simulink library "utility_service_lib"  (Simulink 8.1)
settings: Solver=ode45  StartTime=0.0  StopTime=10.0  RelTol=1e-3
undefined symbols (not defined in the file or in its folder): cable_spec, Left, Ts, type, V
libraries: cables_lib x6, breaker_lib x4, artemis x3, transformer_lib x2, rtlab x1, ssn_lib x1, powerlib x1
settings Model: Creator=RE25624  LastModifiedBy=re25624

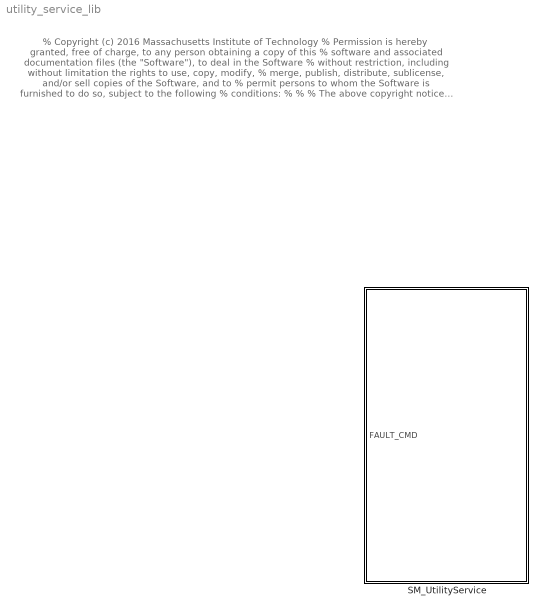
== system utility_service_lib ==
  note: % Copyright (c) 2016 Massachusetts Institute of Technology
      | % Permission is hereby granted, free of charge, to any person obtaining a copy of this
      | % software and associated documentation files (the "Software"), to deal in the Software
      | % without restriction, including without limitation the rights to use, copy, modify,
      | % merge, publish, distribute, sublicense, and/or sell copies of the Software, and to
      | % permit persons to whom the Software is furnished to do so, subject to the following
      | % conditions:
      | %
      | %
      | % The above copyright notice and this permission notice shall be included in
      | % all copies or substantial portions of the Software.
      | %
      | % THE SOFTWARE IS PROVIDED "AS IS", WITHOUT WARRANTY OF ANY KIND, EXPRESS OR IMPLIED,
      | % INCLUDING BUT NOT LIMITED TO THE WARRANTIES OF MERCHANTABILITY, FITNESS FOR A
      | % PARTICULAR PURPOSE AND NONINFRINGEMENT. IN NO EVENT SHALL THE AUTHORS OR COPYRIGHT
      | % HOLDERS BE LIABLE FOR ANY CLAIM, DAMAGES OR OTHER LIABILITY, WHETHER IN AN ACTION
      | % OF CONTRACT, TORT OR OTHERWISE, ARISING FROM, OUT OF OR IN CONNECTION WITH THE
      | % SOFTWARE OR THE USE OR OTHER DEALINGS IN THE SOFTWARE.
      | %
      | %
      | %%
  SM_UtilityService : Subsystem

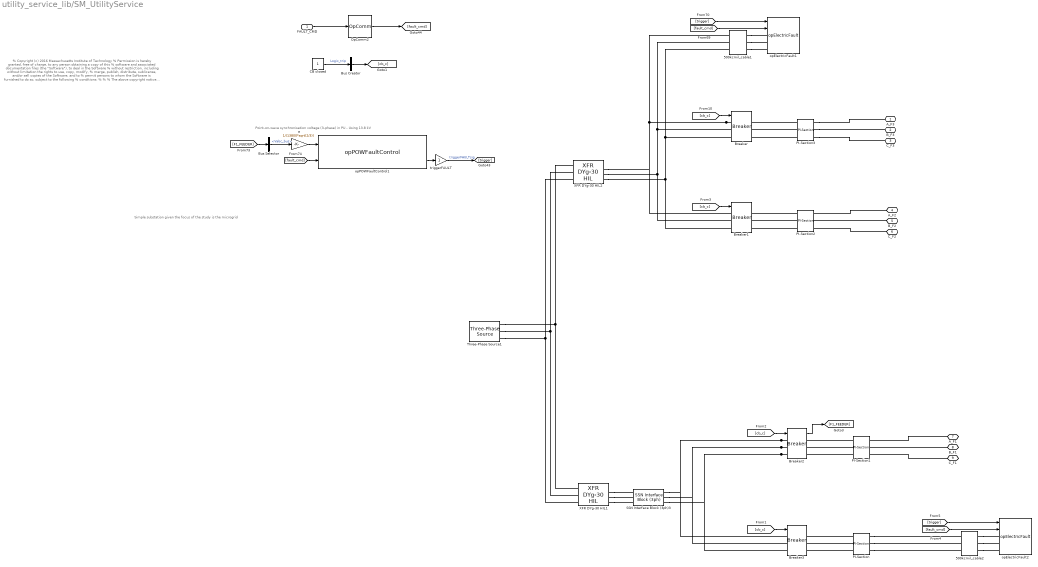
== system utility_service_lib/SM_UtilityService ==
  note: Point-on-wave synchronisation voltage (3-phase) in PU - Using 13.8 kV
  note: % Copyright (c) 2016 Massachusetts Institute of Technology
      | % Permission is hereby granted, free of charge, to any person obtaining a copy of this
      | % software and associated documentation files (the "Software"), to deal in the Software
      | % without restriction, including without limitation the rights to use, copy, modify,
      | % merge, publish, distribute, sublicense, and/or sell copies of the Software, and to
      | % permit persons to whom the Software is furnished to do so, subject to the following
      | % conditions:
      | %
      | %
      | % The above copyright notice and this permission notice shall be included in
      | % all copies or substantial portions of the Software.
      | %
      | % THE SOFTWARE IS PROVIDED "AS IS", WITHOUT WARRANTY OF ANY KIND, EXPRESS OR IMPLIED,
      | % INCLUDING BUT NOT LIMITED TO THE WARRANTIES OF MERCHANTABILITY, FITNESS FOR A
      | % PARTICULAR PURPOSE AND NONINFRINGEMENT. IN NO EVENT SHALL THE AUTHORS OR COPYRIGHT
      | % HOLDERS BE LIABLE FOR ANY CLAIM, DAMAGES OR OTHER LIABILITY, WHETHER IN AN ACTION
      | % OF CONTRACT, TORT OR OTHERWISE, ARISING FROM, OUT OF OR IN CONNECTION WITH THE
      | % SOFTWARE OR THE USE OR OTHER DEALINGS IN THE SOFTWARE.
      | %
      | %
      | %%
  note: Simple substation given the focus of the study is the microgrid
  FAULT_CMD : Inport
  500kcmil_cable1 : cables_lib/500kcmil_cable  length=1  par_sets=1
  500kcmil_cable2 : cables_lib/500kcmil_cable  length=1  par_sets=1
  Breaker{,1..3} (4 alike) : breaker_lib/Breaker  Ts=Ts
  Bus Creator : BusCreator  Inputs=1
  Bus Selector : BusSelector  OutputSignals=Vabc_bus
  CB closed : Constant
  OpComm2 : rtlab/OpComm  nbport=1  groupe_acq=1  subsys_rate=0  st=0  Synchronization=on  Interpolation=on  Threshold=1.0  Missed_Data=off  Sim_Time=off  Samples=off  dynSigOut=off  from_console=1  warning_done=off  writeOpCommFile=off  Offset=off
  PI-Section : cables_lib/PI-Section  cable_spec=[cable_spec(13, :)]  line_length=3000  parallel_sets=1
  PI-Section1 : cables_lib/PI-Section  cable_spec=[cable_spec(13, :)]  line_length=500  parallel_sets=1
  PI-Section2 : cables_lib/PI-Section  cable_spec=[cable_spec(13, :)]  line_length=500  parallel_sets=1
  PI-Section3 : cables_lib/PI-Section  cable_spec=[cable_spec(13, :)]  line_length=500  parallel_sets=1
  SSN Interface Block (3ph)3 : ssn_lib/SSN Interface Block (3ph)  nb_phase=3  nb_port=2  p1_type=V-type(Left)  p2_type=V-type (Right)  p3_type=V-type(Left)  p4_type=V-type(Left)  p5_type=V-type(Left)  p6_type=V-type(Left)  p7_type=V-type(Left)  p8_type=V-type(Left)  p9_type=V-type(Left)  p10_type=V-type(Left)  p11_type=V-type(Left)  p12_type=V-type(Left)  p13_type=V-type(Left)  p14_type=V-type(Left)  p15_type=V-type(Left)  p16_type=V-type(Left)  I_port_shunt_resistance=1e9
  Three-Phase Source1 : powerlib/Electrical Sources/Three-Phase Source  Voltage=115000  PhaseAngle=0  Frequency=60  InternalConnection=Yg  SpecifyImpedance=on  Resistance=0.8929  Inductance=16.58e-3  ShortCircuitLevel=100e6  BaseVoltage=115000  XRratio=30  BusType=swing  Pref=0  Qref=0  Qmin=-inf  Qmax=inf
  XFR DYg-30 HIL1 : transformer_lib/XFR DYg-30 HIL  Rating=50000  Vp=115000  Vs=13800  Z=15  XR=30
  XFR DYg-30 HIL2 : transformer_lib/XFR DYg-30 HIL  Rating=50000  Vp=115000  Vs=13800  Z=15  XR=30
  a : Gain  Gain=1/(13800*sqrt(2/3))
  opElectricFault1 : artemis/Tools /POW faults/opElectricFault  FaultLocation=location 7  FaultResistance=0.0001  GroundResistance=0.0001  InitialStates=[0 0 0]  SnubberResistance=1e6  SnubberCapacitance=inf
  opElectricFault2 : artemis/Tools /POW faults/opElectricFault  FaultLocation=location 8  FaultResistance=0.0001  GroundResistance=0.0001  InitialStates=[0 0 0]  SnubberResistance=1e6  SnubberCapacitance=inf
  opPOWFaultControl1 : artemis/Tools /POW faults/opPOWFaultControl  Ts=Ts  usePLL=off  Fgrid=60  PLL_k=[180 3200 1]  vol_sel=1: rising zero-corssing  SyncPhase_menu=A  T_acq=0.8
  triggerFAULT : Gain
  A_F3 : PMIOPort  Port=1  Side=Right
  B_F3 : PMIOPort  Port=2  Side=Right
  C_F3 : PMIOPort  Port=3  Side=Right
  A_F2 : PMIOPort  Port=4  Side=Right
  B_F2 : PMIOPort  Port=5  Side=Right
  C_F2 : PMIOPort  Port=6  Side=Right
  A_F1 : PMIOPort  Port=7  Side=Right
  B_F1 : PMIOPort  Port=8  Side=Right
  C_F1 : PMIOPort  Port=9  Side=Right
  wires:
  [trigger] -> opElectricFault2/1
  [fault_cmd] -> opElectricFault2/2
  Breaker2/1 -> [F1_FEEDER]
  FAULT_CMD/1 -> OpComm2/1
  OpComm2/1 -> [fault_cmd]
  a/1 -> opPOWFaultControl1/1
  Bus Selector/1 -> a/1  "<Vabc_bus>"
  [F1_FEEDER] -> Bus Selector/1
  triggerFAULT/1 -> [trigger]  "triggerFAULTsig"
  opPOWFaultControl1/2 -> triggerFAULT/1
  [fault_cmd] -> opPOWFaultControl1/2
  [trigger] -> opElectricFault1/1
  [fault_cmd] -> opElectricFault1/2
  CB closed/1 -> Bus Creator/1  "Logic_trip"
  Bus Creator/1 -> [cb_c]
  [cb_c] -> Breaker3/1
  [cb_c] -> Breaker1/1
  [cb_c] -> Breaker/1
  [cb_c] -> Breaker2/1
  connections:
  XFR DYg-30 HIL1/RConn1 -- SSN Interface Block (3ph)3/LConn1
  XFR DYg-30 HIL1/RConn2 -- SSN Interface Block (3ph)3/LConn2
  XFR DYg-30 HIL1/RConn3 -- SSN Interface Block (3ph)3/LConn3
  PI-Section/RConn1 -- 500kcmil_cable2/LConn1
  PI-Section/RConn2 -- 500kcmil_cable2/LConn2
  PI-Section/RConn3 -- 500kcmil_cable2/LConn3
  500kcmil_cable2/RConn1 -- opElectricFault2/LConn1
  500kcmil_cable2/RConn2 -- opElectricFault2/LConn2
  500kcmil_cable2/RConn3 -- opElectricFault2/LConn3
  500kcmil_cable1/RConn1 -- opElectricFault1/LConn1
  500kcmil_cable1/RConn2 -- opElectricFault1/LConn2
  500kcmil_cable1/RConn3 -- opElectricFault1/LConn3
  PI-Section3/RConn2 -- B_F3/RConn1
  C_F1/RConn1 -- PI-Section1/RConn3
  A_F1/RConn1 -- PI-Section1/RConn1
  B_F2/RConn1 -- PI-Section2/RConn2
  PI-Section3/RConn1 -- A_F3/RConn1
  C_F2/RConn1 -- PI-Section2/RConn3
  XFR DYg-30 HIL1/LConn1 -- XFR DYg-30 HIL2/LConn1 -- Three-Phase Source1/RConn1
  XFR DYg-30 HIL1/LConn2 -- XFR DYg-30 HIL2/LConn2 -- Three-Phase Source1/RConn2
  XFR DYg-30 HIL1/LConn3 -- XFR DYg-30 HIL2/LConn3 -- Three-Phase Source1/RConn3
  PI-Section3/RConn3 -- C_F3/RConn1
  B_F1/RConn1 -- PI-Section1/RConn2
  A_F2/RConn1 -- PI-Section2/RConn1
  PI-Section/LConn2 -- Breaker3/RConn2
  XFR DYg-30 HIL2/RConn3 -- Breaker/LConn3 -- 500kcmil_cable1/LConn3 -- Breaker1/LConn3
  Breaker/LConn1 -- 500kcmil_cable1/LConn1 -- Breaker1/LConn1 -- XFR DYg-30 HIL2/RConn1
  XFR DYg-30 HIL2/RConn2 -- Breaker/LConn2 -- 500kcmil_cable1/LConn2 -- Breaker1/LConn2
  PI-Section3/LConn3 -- Breaker/RConn3
  Breaker2/LConn1 -- SSN Interface Block (3ph)3/RConn1 -- Breaker3/LConn1
  PI-Section/LConn1 -- Breaker3/RConn1
  PI-Section2/LConn2 -- Breaker1/RConn2
  PI-Section/LConn3 -- Breaker3/RConn3
  Breaker2/LConn3 -- SSN Interface Block (3ph)3/RConn3 -- Breaker3/LConn3
  PI-Section3/LConn2 -- Breaker/RConn2
  Breaker2/LConn2 -- SSN Interface Block (3ph)3/RConn2 -- Breaker3/LConn2
  PI-Section1/LConn3 -- Breaker2/RConn3
  PI-Section3/LConn1 -- Breaker/RConn1
  PI-Section1/LConn2 -- Breaker2/RConn2
  PI-Section1/LConn1 -- Breaker2/RConn1
  PI-Section2/LConn3 -- Breaker1/RConn3
  PI-Section2/LConn1 -- Breaker1/RConn1
